simulink model "RocketFlightSim"  (R2023b)
settings: Solver=FixedStepAuto  StartTime=0.0  StopTime=30.0  FixedStep=0.01  RelTol=1e-3
libraries: simulink x1
settings Model: Creator=atzml  LastModifiedBy=atzml

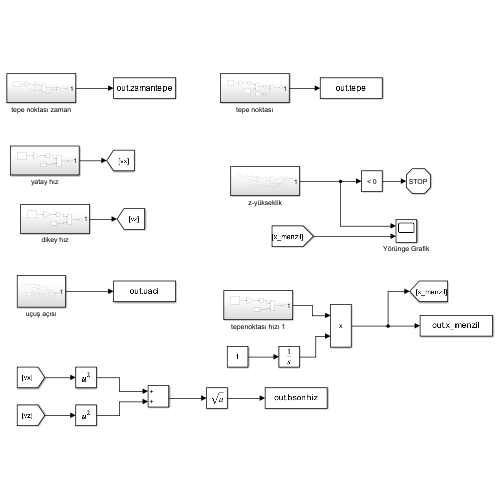
[thumbnail: Simulink's stored preview of the top-level diagram]
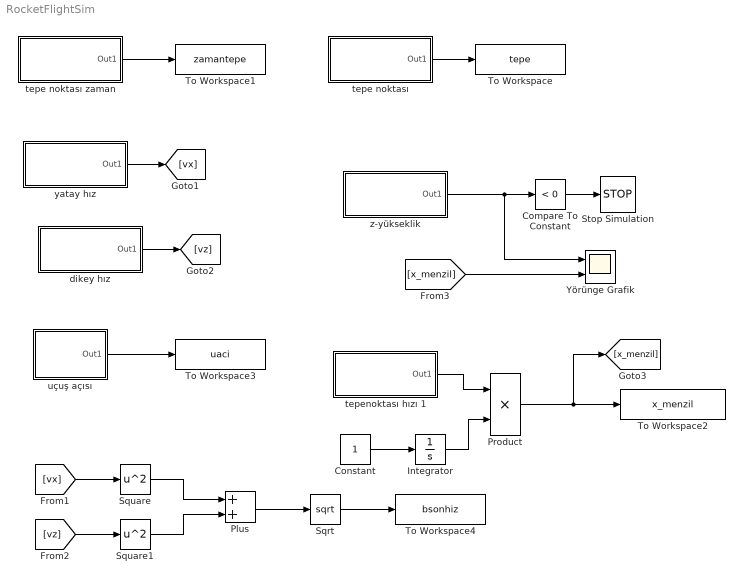
== system RocketFlightSim ==
  Compare To Constant : simulink/Logic and Bit Operations/Compare To Constant  relop=<  const=0  OutDataTypeStr=boolean
  Constant : Constant
  Integrator : Integrator
  Plus : Sum
  Product : Product
  Sqrt : Sqrt
  Square : Math  Operator=square
  Square1 : Math  Operator=square
  Stop Simulation : Stop
  To Workspace : ToWorkspace  VariableName=tepe  SaveFormat=Timeseries  SampleTime=-1
  To Workspace1 : ToWorkspace  VariableName=zamantepe  SaveFormat=Timeseries  SampleTime=-1
  To Workspace2 : ToWorkspace  VariableName=x_menzil  SaveFormat=Timeseries  SampleTime=-1
  To Workspace3 : ToWorkspace  VariableName=uaci  SaveFormat=Timeseries  SampleTime=-1
  To Workspace4 : ToWorkspace  VariableName=bsonhiz  SaveFormat=Timeseries  SampleTime=-1
  Yörünge Grafik : Scope  NumInputPorts=2
  dikey hız : Subsystem
  tepe noktası : Subsystem
  tepe noktası zaman : Subsystem
  tepenoktası hızı 1 : Subsystem
  uçuş açısı : Subsystem
  yatay hız : Subsystem
  z-yükseklik : Subsystem
  wires:
  tepe noktası/1(Out1) -> To Workspace/1
  tepe noktası zaman/1(Out1) -> To Workspace1/1
  tepenoktası hızı 1/1(Out1) -> Product/1
  Product/1 -> [x_menzil], To Workspace2/1
  uçuş açısı/1(Out1) -> To Workspace3/1
  dikey hız/1(Out1) -> [vz]
  Sqrt/1 -> To Workspace4/1
  [vz] -> Square1/1
  Plus/1 -> Sqrt/1
  Square1/1 -> Plus/2
  Square/1 -> Plus/1
  [vx] -> Square/1
  Compare To Constant/1 -> Stop Simulation/1
  z-yükseklik/1(Out1) -> Yörünge Grafik/1, Compare To Constant/1
  Constant/1 -> Integrator/1
  [x_menzil] -> Yörünge Grafik/2
  Integrator/1 -> Product/2
  yatay hız/1(Out1) -> [vx]

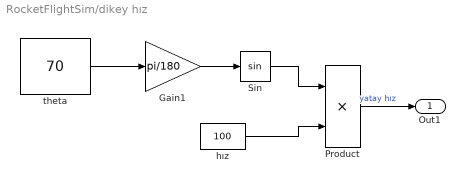
== system RocketFlightSim/dikey hız ==
  Gain1 : Gain  Gain=pi/180
  Product : Product
  Sin : Trigonometry
  hız : Constant  Value=100
  theta : Constant  Value=70
  Out1 : Outport
  wires:
  Product/1 -> Out1/1  "yatay hız"
  Sin/1 -> Product/1
  hız/1 -> Product/2
  Gain1/1 -> Sin/1
  theta/1 -> Gain1/1

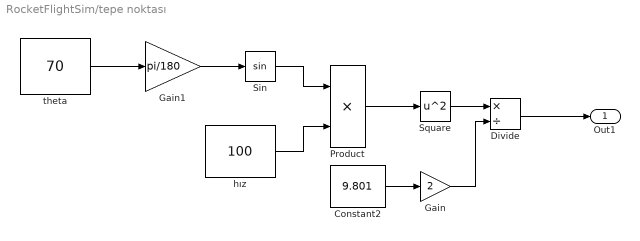
== system RocketFlightSim/tepe noktası ==
  Constant2 : Constant  Value=9.801
  Divide : Product  Inputs=*/
  Gain : Gain  Gain=2
  Gain1 : Gain  Gain=pi/180
  Product : Product
  Sin : Trigonometry
  Square : Math  Operator=square
  hız : Constant  Value=100
  theta : Constant  Value=70
  Out1 : Outport
  wires:
  Sin/1 -> Product/1
  hız/1 -> Product/2
  Product/1 -> Square/1
  Square/1 -> Divide/1
  Constant2/1 -> Gain/1
  Gain/1 -> Divide/2
  Divide/1 -> Out1/1
  theta/1 -> Gain1/1
  Gain1/1 -> Sin/1

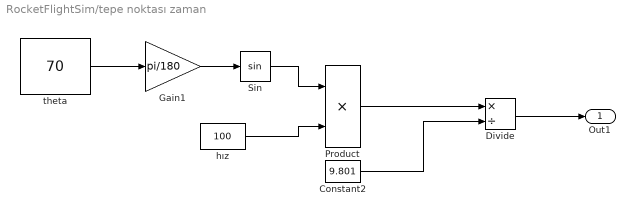
== system RocketFlightSim/tepe noktası zaman ==
  Constant2 : Constant  Value=9.801
  Divide : Product  Inputs=*/
  Gain1 : Gain  Gain=pi/180
  Product : Product
  Sin : Trigonometry
  hız : Constant  Value=100
  theta : Constant  Value=70
  Out1 : Outport
  wires:
  Divide/1 -> Out1/1
  hız/1 -> Product/2
  Product/1 -> Divide/1
  Constant2/1 -> Divide/2
  Sin/1 -> Product/1
  Gain1/1 -> Sin/1
  theta/1 -> Gain1/1

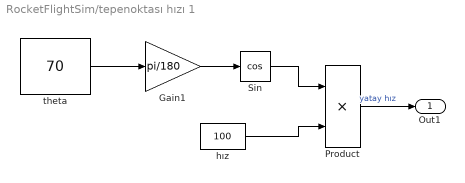
== system RocketFlightSim/tepenoktası hızı 1 ==
  Gain1 : Gain  Gain=pi/180
  Product : Product
  Sin : Trigonometry  Operator=cos
  hız : Constant  Value=100
  theta : Constant  Value=70
  Out1 : Outport
  wires:
  theta/1 -> Gain1/1
  Gain1/1 -> Sin/1
  hız/1 -> Product/2
  Sin/1 -> Product/1
  Product/1 -> Out1/1  "yatay hız"

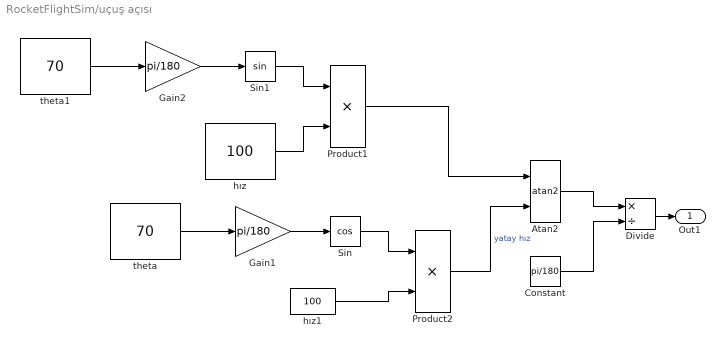
== system RocketFlightSim/uçuş açısı ==
  Atan2 : Trigonometry  Operator=atan2
  Constant : Constant  Value=pi/180
  Divide : Product  Inputs=*/
  Gain1 : Gain  Gain=pi/180
  Gain2 : Gain  Gain=pi/180
  Product1 : Product
  Product2 : Product
  Sin : Trigonometry  Operator=cos
  Sin1 : Trigonometry
  hız : Constant  Value=100
  hız1 : Constant  Value=100
  theta : Constant  Value=70
  theta1 : Constant  Value=70
  Out1 : Outport
  wires:
  Atan2/1 -> Divide/1
  theta/1 -> Gain1/1
  Sin1/1 -> Product1/1
  hız1/1 -> Product2/2
  Gain2/1 -> Sin1/1
  theta1/1 -> Gain2/1
  Gain1/1 -> Sin/1
  Sin/1 -> Product2/1
  hız/1 -> Product1/2
  Product1/1 -> Atan2/1
  Constant/1 -> Divide/2
  Product2/1 -> Atan2/2  "yatay hız"
  Divide/1 -> Out1/1

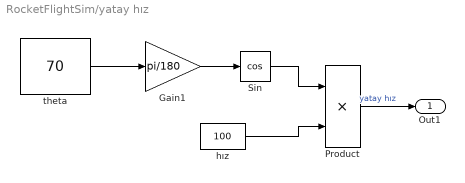
== system RocketFlightSim/yatay hız ==
  Gain1 : Gain  Gain=pi/180
  Product : Product
  Sin : Trigonometry  Operator=cos
  hız : Constant  Value=100
  theta : Constant  Value=70
  Out1 : Outport
  wires:
  Product/1 -> Out1/1  "yatay hız"
  Sin/1 -> Product/1
  hız/1 -> Product/2
  Gain1/1 -> Sin/1
  theta/1 -> Gain1/1

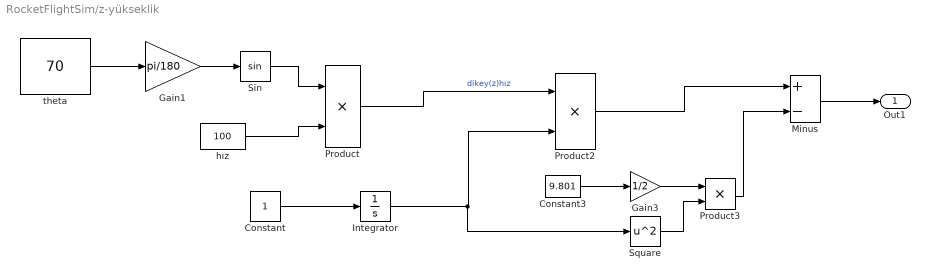
== system RocketFlightSim/z-yükseklik ==
  Constant : Constant
  Constant3 : Constant  Value=9.801
  Gain1 : Gain  Gain=pi/180
  Gain3 : Gain  Gain=1/2
  Integrator : Integrator
  Minus : Sum  Inputs=+-
  Product : Product
  Product2 : Product
  Product3 : Product
  Sin : Trigonometry
  Square : Math  Operator=square
  hız : Constant  Value=100
  theta : Constant  Value=70
  Out1 : Outport
  wires:
  Product/1 -> Product2/1  "dikey(z)hız"
  Sin/1 -> Product/1
  hız/1 -> Product/2
  Gain1/1 -> Sin/1
  theta/1 -> Gain1/1
  Constant3/1 -> Gain3/1
  Integrator/1 -> Square/1, Product2/2
  Square/1 -> Product3/2
  Gain3/1 -> Product3/1
  Product3/1 -> Minus/2
  Product2/1 -> Minus/1
  Constant/1 -> Integrator/1
  Minus/1 -> Out1/1
